simulink model "regolatore_1"  (R2022b)
settings: Solver=VariableStepAuto  StartTime=0.0  StopTime=20  RelTol=1e-3
libraries: robotmobilelib x1
settings Model: Creator=thoma  LastModifiedBy=thoma

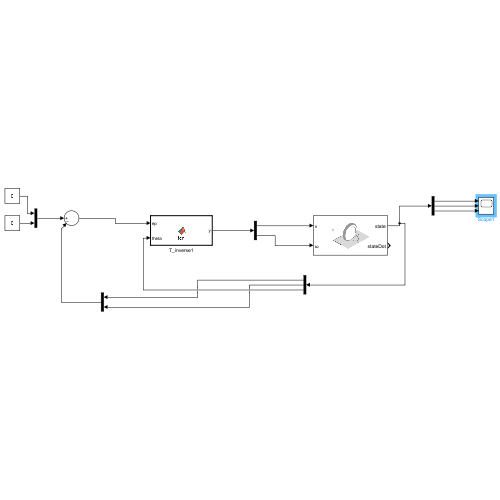
[thumbnail: Simulink's stored preview of the top-level diagram]
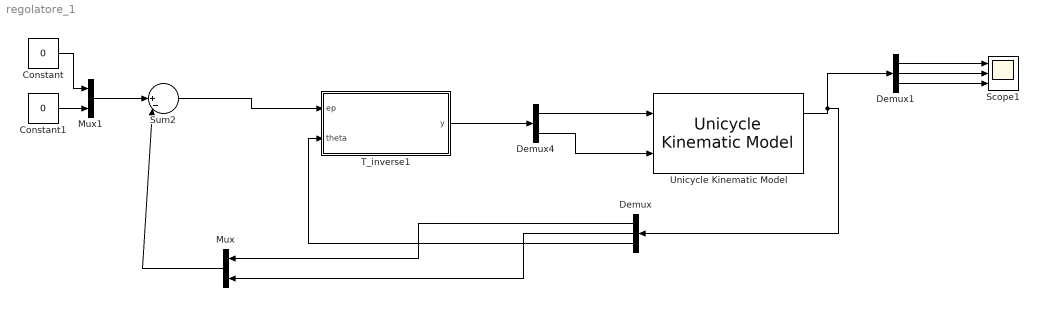
== system regolatore_1 ==
  Constant : Constant  Value=0
  Constant1 : Constant  Value=0
  Demux : Demux  Outputs=3
  Demux1 : Demux  Outputs=3
  Demux4 : Demux  Outputs=2
  Mux : Mux  Inputs=2
  Mux1 : Mux  Inputs=2
  Scope1 : Scope  NumInputPorts=3
  Sum2 : Sum  Inputs=||+-|
  T_inverse1 : MATLAB Function  TreatAsAtomicUnit=on
  Unicycle Kinematic Model : robotmobilelib/Unicycle Kinematic Model  VehicleInputs=Vehicle Speed & Heading Angular Velocity  WheelRadius=2  WheelSpeedRange=[-Inf Inf]  InitialState=[0;0;0]  SimulateUsing=Interpreted execution
  wires:
  Sum2/1 -> T_inverse1/1(ep)
  Unicycle Kinematic Model/1 -> Demux1/1, Demux/1
  T_inverse1/1(y) -> Demux4/1
  Demux/3 -> T_inverse1/2(theta)
  Demux/2 -> Mux/2
  Demux/1 -> Mux/1
  Mux/1 -> Sum2/2
  Constant1/1 -> Mux1/2
  Constant/1 -> Mux1/1
  Mux1/1 -> Sum2/1
  Demux4/1 -> Unicycle Kinematic Model/1
  Demux4/2 -> Unicycle Kinematic Model/2
  Demux1/1 -> Scope1/1
  Demux1/2 -> Scope1/2
  Demux1/3 -> Scope1/3

== matlab function regolatore_1/T_inverse1 ==
  data: ep input; y output; theta input
function y = fcn(ep,theta)
theta=mod(theta+pi,2*pi)-pi;
kv=2;
kw=6;
v=kv*(ep(1)*cos(theta)+ep(2)*sin(theta));
w=kw*(atan2(-ep(2),-ep(1))+pi-theta);
y = [v;w];
